simulink model "test_senddq"  (Simulink 7.9)
settings: Solver=ode45  StartTime=0.0  StopTime=inf  RelTol=1e-3
libraries: simulink_extras x2, WBCLibrary x2
settings Model: Creator=jorhabib  LastModifiedBy=daniele

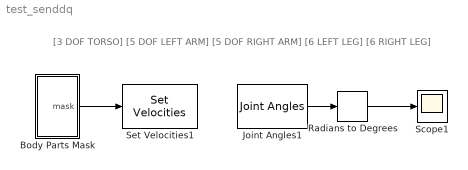
== system test_senddq ==
  note: [3 DOF TORSO] [5 DOF LEFT ARM] [5 DOF RIGHT ARM] [6 LEFT LEG] [6 RIGHT LEG]
  Body Parts Mask : Subsystem
  Joint Angles1 : WBCLibrary/wholeBodyStates/Joint Angles  robotName=robotName  localName=localName
  Radians to Degrees : simulink_extras/Transformations/Radians to Degrees
  Scope1 : Scope
      settings: YMin=-50  YMax=50
  Set Velocities1 : WBCLibrary/wholeBodyActuators/Set Velocities  val=4  robotName=robotName  localName=localName
  wires:
  Joint Angles1/1 -> Radians to Degrees/1
  Radians to Degrees/1 -> Scope1/1
  Body Parts Mask/1(mask) -> Set Velocities1/1

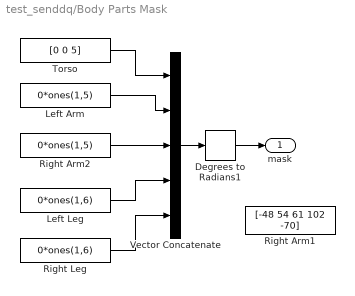
== system test_senddq/Body Parts Mask ==
  Degrees to Radians1 : simulink_extras/Transformations/Degrees to Radians
  Left Arm : Constant  Value=0*ones(1,5)  VectorParams1D=off
  Left Leg : Constant  Value=0*ones(1,6)  VectorParams1D=off
  Right Arm1 : Constant  Value=[-48 54 61 102 -70]  VectorParams1D=off
  Right Arm2 : Constant  Value=0*ones(1,5)  VectorParams1D=off
  Right Leg : Constant  Value=0*ones(1,6)  VectorParams1D=off
  Torso : Constant  Value=[0 0 5]  VectorParams1D=off
  Vector Concatenate : Concatenate  NumInputs=5
  mask : Outport
  wires:
  Torso/1 -> Vector Concatenate/1
  Left Arm/1 -> Vector Concatenate/2
  Right Arm2/1 -> Vector Concatenate/3
  Left Leg/1 -> Vector Concatenate/4
  Right Leg/1 -> Vector Concatenate/5
  Vector Concatenate/1 -> Degrees to Radians1/1
  Degrees to Radians1/1 -> mask/1
